simulink model "simulProjet"  (R2020a)
settings: Solver=VariableStepAuto  StartTime=0.0  StopTime=Tsim  RelTol=1e-3
values from neighbouring files (symbols this model uses):
  Te = 1/Fe    (= 3.125e-06)    [projet.m]    (also in script.m = 0.0111607142857)
  Tsim = T - Te    (= 0.000196875)    [projet.m]    (also in script.m = 0.345982142857)
settings Model: Creator=imbergam  LastModifiedBy=imbergam

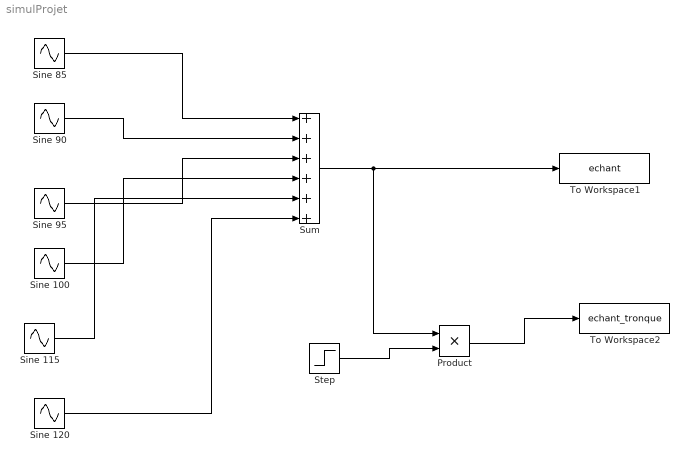
== system simulProjet ==
  Product : Product
  Sine 100 : Sin  Frequency=2*pi*100e3  SampleTime=0
  Sine 115 : Sin  Frequency=2*pi*115e3  SampleTime=0
  Sine 120 : Sin  Frequency=2*pi*120e3  SampleTime=0
  Sine 85 : Sin  Frequency=2*pi*85e3  SampleTime=0
  Sine 90 : Sin  Frequency=2*pi*90e3  SampleTime=0
  Sine 95 : Sin  Frequency=2*pi*95e3  SampleTime=0
  Step : Step  Time=Tsim/2  SampleTime=0
  Sum : Sum  Inputs=++++++
  To Workspace1 : ToWorkspace  VariableName=echant  SaveFormat=Timeseries  SampleTime=Te
  To Workspace2 : ToWorkspace  VariableName=echant_tronque  SaveFormat=Timeseries  SampleTime=Te
  wires:
  Sine 85/1 -> Sum/1
  Sine 90/1 -> Sum/2
  Sine 95/1 -> Sum/3
  Sine 100/1 -> Sum/4
  Sine 115/1 -> Sum/5
  Sine 120/1 -> Sum/6
  Sum/1 -> Product/1, To Workspace1/1
  Step/1 -> Product/2
  Product/1 -> To Workspace2/1
